simulink model "Parqueadero"  (R2020b)
settings: Solver=VariableStepAuto  StartTime=0.0  StopTime=inf  RelTol=1e-3
settings Model: Creator=mateo  LastModifiedBy=mateo
settings OptimizationCC: DefaultParameterBehavior=Inlined  UseDivisionForNetSlopeComputation=on  GainParamInheritBuiltInType=on  UseFloatMulNetSlope=on  InlineInvariantSignals=on  PassReuseOutputArgsAs=Individual arguments  ZeroExternalMemoryAtStartup=off  ZeroInternalMemoryAtStartup=off  NoFixptDivByZeroProtection=on  EfficientFloat2IntCast=on  LifeSpan=1  OptimizeBlockOrder=speed  DifferentSizesBufferReuse=on  EfficientTunableParamExpr=on
settings DebuggingCC: ParameterTunabilityLossMsg=error
settings HardwareCC: ProdLongLongMode=on
settings SFSimCC: MATLABDynamicMemAlloc=off
settings RTWCC: Description=Embedded Coder  SystemTargetFile=ert.tlc  TemplateMakefile=ert_default_tmf  GenerateReport=on  LaunchReport=on  GenerateWebview=on
settings CodeAppCC: ForceParamTrailComments=on  IgnoreCustomStorageClasses=off  OperatorAnnotations=on  SimulinkDataObjDesc=on  SFDataObjDesc=on  CustomSymbolStrGlobalVar=rt$N$M  CustomSymbolStrType=$N$M  CustomSymbolStrFcn=$N$M$F  CustomSymbolStrMacro=$N$M  InsertBlockDesc=on
settings ERTTargetCC: TargetLangStandard=C99 (ISO)  GenerateSampleERTMain=on  IncludeMdlTerminateFcn=off  CombineSignalStateStructs=on  SupportComplex=off  SupportContinuousTime=on  SupportNonInlinedSFcns=on  InlinedParameterPlacement=NonHierarchical  ERTCustomFileTemplate=example_file_process.tlc  ERTFilePackagingFormat=CompactWithDataFile

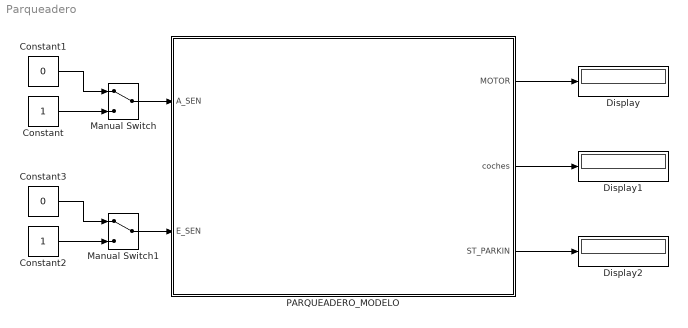
== system Parqueadero ==
  Constant : Constant
  Constant1 : Constant  Value=0
  Constant2 : Constant
  Constant3 : Constant  Value=0
  Display : Display
  Display1 : Display
  Display2 : Display
  Manual Switch : ManualSwitch
  Manual Switch1 : ManualSwitch
  "PARQUEADERO_MODELO " : Subsystem
  wires:
  Constant1/1 -> Manual Switch/1
  Constant/1 -> Manual Switch/2
  Constant2/1 -> Manual Switch1/2
  Constant3/1 -> Manual Switch1/1
  Manual Switch/1 -> "PARQUEADERO_MODELO "/1(A_SEN)
  Manual Switch1/1 -> "PARQUEADERO_MODELO "/2(E_SEN)
  "PARQUEADERO_MODELO "/1(MOTOR) -> Display/1
  "PARQUEADERO_MODELO "/2(coches) -> Display1/1
  "PARQUEADERO_MODELO "/3(ST_PARKIN) -> Display2/1

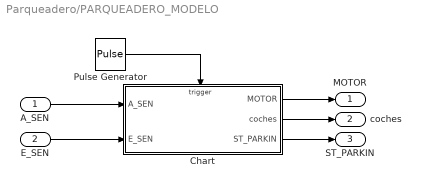
== system Parqueadero/PARQUEADERO_MODELO  ==
  A_SEN : Inport
  E_SEN : Inport  Port=2
  Chart : Stateflow chart  TreatAsAtomicUnit=on
  Pulse Generator : DiscretePulseGenerator  PulseType=Time based  Period=0.1  PulseWidth=5
  MOTOR : Outport
  coches : Outport  Port=2
  ST_PARKIN : Outport  Port=3
  wires:
  Chart/2(coches) -> coches/1
  Pulse Generator/1 -> Chart/Trigger
  Chart/3(ST_PARKIN) -> ST_PARKIN/1
  A_SEN/1 -> Chart/1(A_SEN)
  Chart/1(MOTOR) -> MOTOR/1
  E_SEN/1 -> Chart/2(E_SEN)

== stateflow chart Parqueadero/PARQUEADERO_MODELO /Chart ==
  state inicio_
    entry:
    numero_coches=0;
    coches=0;
    MOTOR=0;
    ST_PARKIN=1;
    ON_OFF=1;
  state OCUPADO
    state inicio
      entry:
      ST_PARKIN=0;
      MOTOR=0;
    state RESTAR_COCHES
      entry:
      numero_coches=numero_coches-1;
      coches=numero_coches;
    state PASO_LIBRE
      entry:
      ON_OFF=1;
    (default) -> OCUPADO.inicio
    OCUPADO.inicio -> OCUPADO.RESTAR_COCHES : [E_SEN==1]
    OCUPADO.RESTAR_COCHES -> PASO_LIBRE : [E_SEN==0]
  state LIBRE
    state inicio
      entry:
      ST_PARKIN=0;
      MOTOR=0;
    state RESTAR_COCHES
      entry:
      numero_coches=numero_coches-1;
      coches=numero_coches;
    state SUMAR_COCHES1
      entry:
      numero_coches=numero_coches+1;
      coches=numero_coches;
      MOTOR=1;
    state CERRAR_PUERTA
      entry:
      MOTOR=0;
    state paso_ocupado
      entry:
      ON_OFF=0;
    LIBRE.RESTAR_COCHES -> LIBRE.inicio : [E_SEN==0]
    (default) -> LIBRE.inicio
    LIBRE.inicio -> LIBRE.RESTAR_COCHES [order 1] : [E_SEN==1]
    CERRAR_PUERTA -> LIBRE.inicio [order 2]
    LIBRE.inicio -> SUMAR_COCHES1 [order 2] : [A_SEN==1]
    SUMAR_COCHES1 -> CERRAR_PUERTA : [A_SEN==0]
    CERRAR_PUERTA -> paso_ocupado [order 1] : [numero_coches==10]
  (default) -> inicio_
  LIBRE -> OCUPADO : [ON_OFF==0]
  inicio_ -> LIBRE
  OCUPADO -> LIBRE : [ON_OFF==1]
  data: A_SEN input; E_SEN input; MOTOR output; coches output; numero_coches local; ST_PARKIN output; ON_OFF local
  events: CLOCK input EITHER_EDGE_EVENT
